simulink model "FM_SIM"  (R2024a)
settings: Solver=VariableStepAuto  StartTime=0.0  StopTime=10.0  RelTol=1e-3
settings Model: Creator=adity  LastModifiedBy=adity

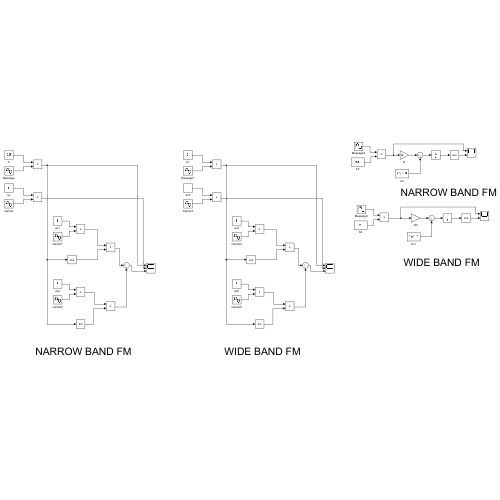
[thumbnail: Simulink's stored preview of the top-level diagram]
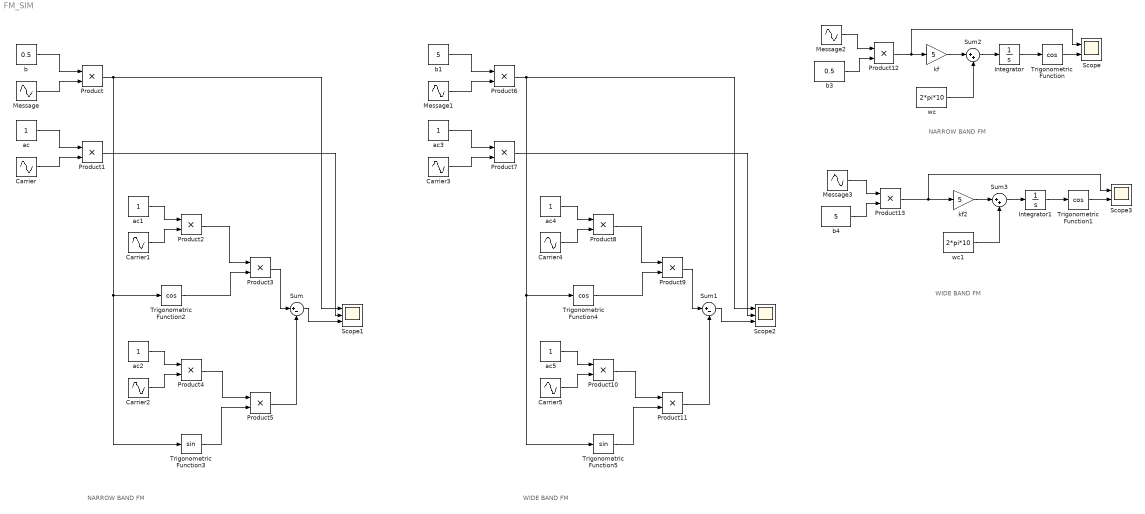
== system FM_SIM ==
  note: NARROW BAND FM
  note: WIDE BAND FM
  note: WIDE BAND FM
  note: NARROW BAND FM
  Carrier{,1,3..4} (4 alike) : Sin  Frequency=2*pi*10  Phase=pi/2  SampleTime=1/1000
  Carrier2 : Sin  Frequency=2*pi*10  SampleTime=1/1000
  Carrier5 : Sin  Frequency=2*pi*10  SampleTime=1/1000
  Integrator : Integrator
  Integrator1 : Integrator
  Message{,1..3} (4 alike) : Sin  Frequency=2*pi*1  SampleTime=1/1000
  Product{,1..13} (14 alike) : Product
  Scope : Scope  NumInputPorts=2
  Scope1 : Scope  NumInputPorts=3
  Scope2 : Scope  NumInputPorts=3
  Scope3 : Scope  NumInputPorts=2
  Sum : Sum  Inputs=|+-
  Sum1 : Sum  Inputs=|+-
  Sum2 : Sum  Inputs=|++
  Sum3 : Sum  Inputs=|++
  Trigonometric Function{,1..2,4} (4 alike) : Trigonometry  Operator=cos
  Trigonometric Function3 : Trigonometry
  Trigonometric Function5 : Trigonometry
  ac{,1..5} (6 alike) : Constant
  b : Constant  Value=0.5
  b1 : Constant  Value=5
  b3 : Constant  Value=0.5
  b4 : Constant  Value=5
  kf : Gain  Gain=5
  kf2 : Gain  Gain=5
  wc : Constant  Value=2*pi*10
  wc1 : Constant  Value=2*pi*10
  wires:
  kf/1 -> Sum2/1
  kf2/1 -> Sum3/1
  wc/1 -> Sum2/2
  Carrier3/1 -> Product7/2
  Product13/1 -> Scope3/1, kf2/1
  Product/1 -> Scope1/1, Trigonometric Function3/1, Trigonometric Function2/1
  ac/1 -> Product1/1
  b/1 -> Product/1
  Product5/1 -> Sum/2
  b4/1 -> Product13/2
  Carrier1/1 -> Product2/2
  ac2/1 -> Product4/1
  Product2/1 -> Product3/1
  Trigonometric Function2/1 -> Product3/2
  ac1/1 -> Product2/1
  Sum1/1 -> Scope2/3
  Integrator/1 -> Trigonometric Function/1
  Product1/1 -> Scope1/2
  Sum/1 -> Scope1/3
  Message/1 -> Product/2
  Product4/1 -> Product5/1
  Product6/1 -> Scope2/1, Trigonometric Function5/1, Trigonometric Function4/1
  Product12/1 -> Scope/1, kf/1
  Trigonometric Function5/1 -> Product11/2
  Carrier5/1 -> Product10/2
  Product3/1 -> Sum/1
  ac3/1 -> Product7/1
  b1/1 -> Product6/1
  Message3/1 -> Product13/1
  Product11/1 -> Sum1/2
  Sum2/1 -> Integrator/1
  Product7/1 -> Scope2/2
  Trigonometric Function3/1 -> Product5/2
  Product9/1 -> Sum1/1
  Carrier/1 -> Product1/2
  Trigonometric Function/1 -> Scope/2
  Trigonometric Function1/1 -> Scope3/2
  Carrier2/1 -> Product4/2
  Product10/1 -> Product11/1
  Integrator1/1 -> Trigonometric Function1/1
  Sum3/1 -> Integrator1/1
  Message2/1 -> Product12/1
  wc1/1 -> Sum3/2
  ac4/1 -> Product8/1
  ac5/1 -> Product10/1
  Product8/1 -> Product9/1
  Message1/1 -> Product6/2
  Carrier4/1 -> Product8/2
  b3/1 -> Product12/2
  Trigonometric Function4/1 -> Product9/2
